simulink model "ex5_StateChart1"  (R2024a)
settings: Solver=FixedStepDiscrete  StartTime=0.0  StopTime=20.0  FixedStep=0.1  RelTol=1e-3  EnableMultiTasking=on
settings Model: PacingRate=0.500000  ExtModeTrigDuration=2  Creator=erfuu  LastModifiedBy=erfuu
settings SolverCC: AlgebraicLoopSolver=TrustRegion  AutoInsertRateTranBlk=on
settings DataIOCC: LimitDataPoints=on
settings OptimizationCC: EnhancedBackFolding=on  PassReuseOutputArgsAs=Individual arguments  ZeroExternalMemoryAtStartup=off  ZeroInternalMemoryAtStartup=off  MaxStackSize=64  OptimizeBlockOrder=speed  DifferentSizesBufferReuse=on  OptimizationCustomize=off  EfficientTunableParamExpr=on
settings DebuggingCC: ParameterTunabilityLossMsg=error  UnconnectedInputMsg=warning  UnconnectedOutputMsg=warning  UnconnectedLineMsg=warning  AllowSymbolicDim=off  SFUnexpectedBacktrackingDiag=warning  SFNoUnconditionalDefaultTransitionDiag=warning  SFExecutionAtInitializationDiag=none  ArithmeticOperatorsInVariantConditions=warning
settings HardwareCC: ProdBitPerInt=16  ProdBitPerPointer=16  ProdBitPerSizeT=16  ProdBitPerPtrDiffT=16  ProdLargestAtomicFloat=None  ProdWordSize=8  ProdHWDeviceType=Atmel->AVR
settings ModelReferenceCC: EnableRefExpFcnMdlSchedulingChecks=on
settings SFSimCC: SimUseLocalCustomCode=off  MATLABDynamicMemAlloc=off  CustomCodeUndefinedFunction=UseInterfaceOnly
settings RTWCC: Description=Embedded Coder  SystemTargetFile=ert.tlc  HardwareBoard=Arduino Mega 2560  TemplateMakefile=ert_default_tmf  RTWUseLocalCustomCode=off  Toolchain=Arduino AVR  BuildConfiguration=Faster Runs  GPUComputeCapability=3.5  DLArmComputeVersion=19.05
settings CodeAppCC: ForceParamTrailComments=on  IgnoreCustomStorageClasses=off  OperatorAnnotations=on  SimulinkDataObjDesc=on  SFDataObjDesc=on  InsertBlockDesc=on
settings ERTTargetCC: SupportContinuousTime=on  SupportVariableSizeSignals=on  ExtModeTransport=3  ExtModeStaticAlloc=on  ExtModeAutomaticAllocSize=off  ExtModeStaticAllocSize=2048  ExtModeMexFile=ext_xcp  ExtModeIntrfLevel=Level2 - Open
settings ConfigComp: CovMetricSettings=dw  CovSaveCumulativeToWorkspaceVar=on  CovSaveSingleToWorkspaceVar=on  CovExternalEMLEnable=off

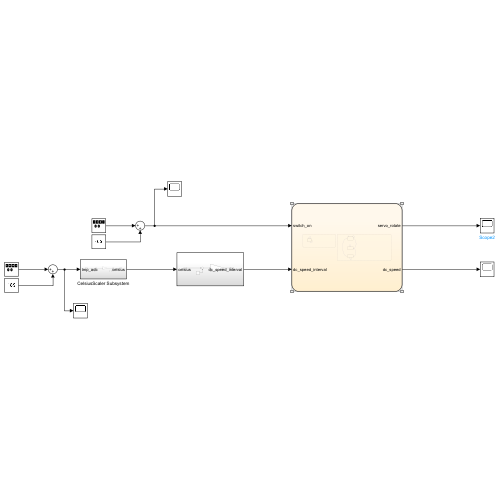
[thumbnail: Simulink's stored preview of the top-level diagram]
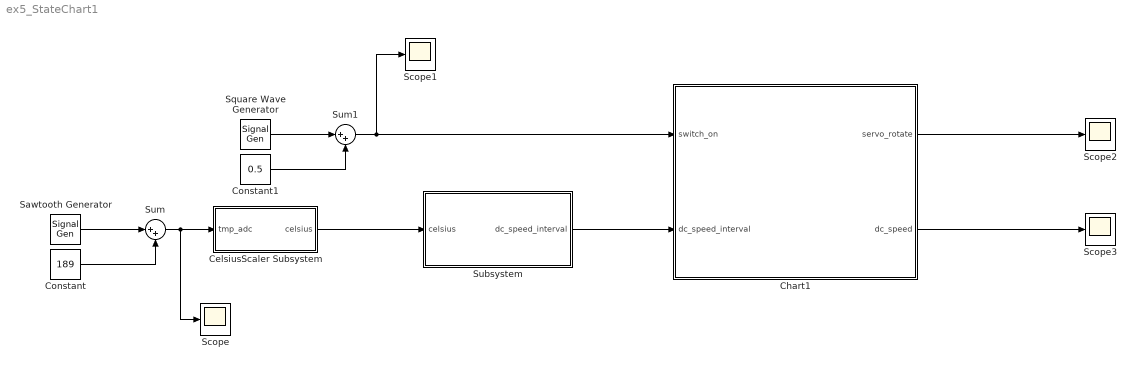
== system ex5_StateChart1 ==
  CelsiusScaler Subsystem : Subsystem
  Chart1 : Stateflow chart  TreatAsAtomicUnit=on
  Constant : Constant  Value=189
  Constant1 : Constant  Value=0.5
  Sawtooth Generator : SignalGenerator  WaveForm=sawtooth  Amplitude=169  Frequency=0.25
  Scope{,1..3} (4 alike) : Scope
  Square Wave Generator : SignalGenerator  WaveForm=square  Amplitude=0.5  Frequency=0.5
  Subsystem : Subsystem
  Sum : Sum  Inputs=|++
  Sum1 : Sum  Inputs=|++
  wires:
  Chart1/1(servo_rotate) -> Scope2/1
  Chart1/2(dc_speed) -> Scope3/1
  Sum/1 -> Scope/1, CelsiusScaler Subsystem/1(tmp_adc)
  Sawtooth Generator/1 -> Sum/1
  Constant/1 -> Sum/2
  Square Wave Generator/1 -> Sum1/1
  Sum1/1 -> Scope1/1, Chart1/1(switch_on)
  Constant1/1 -> Sum1/2
  CelsiusScaler Subsystem/1(celsius) -> Subsystem/1(celsius)
  Subsystem/1(dc_speed_interval) -> Chart1/2(dc_speed_interval)

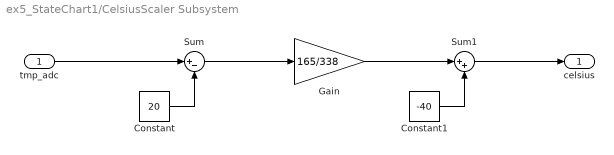
== system ex5_StateChart1/CelsiusScaler Subsystem ==
  tmp_adc : Inport
  Constant : Constant  Value=20
  Constant1 : Constant  Value=-40
  Gain : Gain  Gain=165/338
  Sum : Sum  Inputs=|+-
  Sum1 : Sum  Inputs=|++
  celsius : Outport
  wires:
  Constant/1 -> Sum/2
  tmp_adc/1 -> Sum/1
  Constant1/1 -> Sum1/2
  Gain/1 -> Sum1/1
  Sum1/1 -> celsius/1
  Sum/1 -> Gain/1

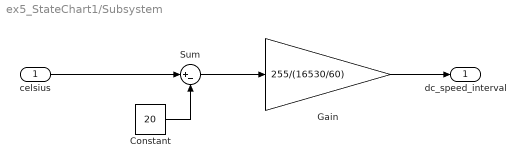
== system ex5_StateChart1/Subsystem ==
  celsius : Inport
  Constant : Constant  Value=20
  Gain : Gain  Gain=255/(16530/60)
  Sum : Sum  Inputs=|+-
  dc_speed_interval : Outport
  wires:
  Constant/1 -> Sum/2
  celsius/1 -> Sum/1
  Sum/1 -> Gain/1
  Gain/1 -> dc_speed_interval/1

== stateflow chart ex5_StateChart1/Chart1 ==
  state DC_Motor [parallel]
    settings: executionOrder=2
    state check
    check -> check [order 1] : [ctr_dc < (DC_PERIOD / STEP_SIZE) - 1]{ctr_dc = ctr_dc + 1}
    (default) -> check
    check -> check [order 2] : [ctr_dc >= (DC_PERIOD / STEP_SIZE) - 1]{dc_speed = dc_speed_interval; ctr_dc = 0;}
  state Servo_Motor [parallel]
    settings: executionOrder=1
    state Natural
    state ClockWise
    state Counter_ClockWise
    (default) -> Natural
    Natural -> Natural [order 2] : [ctr_servo < ((SLOW_MODE_DURATION - (switch_on * (SLOW_MODE_DURATION - FAST_MODE_DURATION))) / STEP_SIZE) - 1]{ctr_servo = ctr_servo + 1}
    Counter_ClockWise -> Natural [order 2] : [ctr_servo >= (SERVO_MAX_ANGLE / SERVO_ANGLE_CHANGE) - 1]{servo_rotate = 0; ctr_servo = 0}
    Natural -> ClockWise [order 1] : [ctr_servo >= ((SLOW_MODE_DURATION - (switch_on * (SLOW_MODE_DURATION - FAST_MODE_DURATION))) / STEP_SIZE) - 1]{servo_rotate = 1; ctr_servo = 0}
    ClockWise -> ClockWise [order 2] : [ctr_servo < (SERVO_MAX_ANGLE / SERVO_ANGLE_CHANGE) - 1]{ctr_servo = ctr_servo + 1}
    ClockWise -> Counter_ClockWise [order 1] : [ctr_servo >= (SERVO_MAX_ANGLE / SERVO_ANGLE_CHANGE) - 1]{servo_rotate = -1; ctr_servo = 0}
    Counter_ClockWise -> Counter_ClockWise [order 1] : [ctr_servo < (SERVO_MAX_ANGLE / SERVO_ANGLE_CHANGE) - 1]{ctr_servo = ctr_servo + 1}
  data: SLOW_MODE_DURATION constant uint16 =10000; servo_rotate output int16 =0; FAST_MODE_DURATION constant uint16 =5000; STEP_SIZE constant uint16 =100; switch_on input; ctr_dc local uint16 =0; ctr_servo local uint16 =0; SERVO_MAX_ANGLE constant uint16 =180; SERVO_ANGLE_CHANGE constant uint16 =10; DC_PERIOD constant uint16 =1000; dc_speed output =0; dc_speed_interval input
